simulink model "simulinkdelsistema"  (R2026a)
settings: Solver=VariableStepAuto  StopTime=15
settings Model: Creator=Andru Fonseca  LastModifiedBy=Andru Fonseca

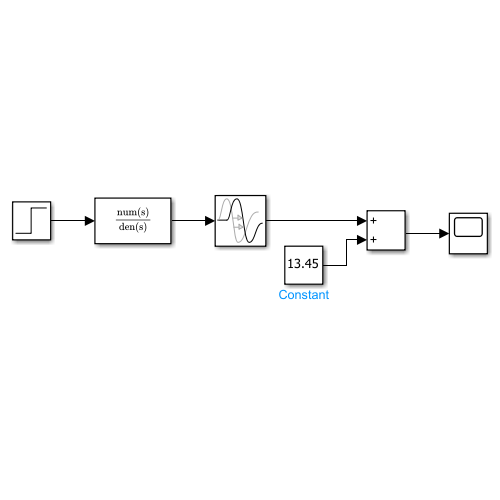
[thumbnail: Simulink's stored preview of the top-level diagram]
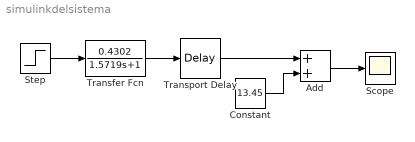
== system simulinkdelsistema ==
  Add : Sum
  Constant : Constant  Value=13.45
  Scope : Scope
      settings: ActiveDisplayYMinimum=10.761640256281645  ActiveDisplayYMaximum=37.645237693465212
  Step : Step  FinalValue=50  SampleTime=0
  Transfer Fcn : TransferFcn  Numerator=[0.4302]  Denominator=[1.5719 1]
  Transport Delay : TransportDelay  DelayTime=0.1188
  wires:
  Step/1 -> Transfer Fcn/1
  Transfer Fcn/1 -> Transport Delay/1
  Transport Delay/1 -> Add/1
  Add/1 -> Scope/1
  Constant/1 -> Add/2
